simulink model "SIFT-Sysgen"  (R2013a)
settings: Solver=FixedStepDiscrete  SolverMode=SingleTasking  StartTime=0.0  StopTime=10.0  RelTol=1e-3
libraries: xbsIndex_r4 x365, xrbsImage_r4 x64
(part 3 of 10)

== system SIFT-Sysgen/Window Generator ==
  In1 : Inport
  Delay{,1..5} (6 alike) : xbsIndex_r4/Delay  rst=off  infoeditControl=Selection of Reset will increase slice count due to use of real FFs and instead of SRLs  en=off  latency=1  dbl_ovrd=off  reg_retiming=off  block_type=delay
  Virtex Line Buffer : xrbsImage_r4/Virtex Line Buffer  buf_depth=1200  cst=1
  Virtex Line Buffer1 : xrbsImage_r4/Virtex Line Buffer  buf_depth=1200  cst=1
  Out1 : Outport
  Out2 : Outport  Port=2
  Out3 : Outport  Port=3
  Out4 : Outport  Port=4
  Out5 : Outport  Port=5
  Out6 : Outport  Port=6
  Out7 : Outport  Port=7
  Out8 : Outport  Port=8
  Out9 : Outport  Port=9
  wires:
  In1/1 -> Out1/1, Delay/1
  Delay/1 -> Out2/1, Delay1/1
  Delay4/1 -> Out8/1, Delay5/1
  Delay2/1 -> Out5/1, Delay3/1
  Virtex Line Buffer/1 -> Delay4/1, Out7/1
  Virtex Line Buffer1/1 -> Out4/1, Delay2/1
  Delay1/1 -> Virtex Line Buffer1/1, Out3/1
  Delay3/1 -> Virtex Line Buffer/1, Out6/1
  Delay5/1 -> Out9/1

== system SIFT-Sysgen/Window Generator1 ==
  In1 : Inport
  Delay{,1..5} (6 alike) : xbsIndex_r4/Delay  rst=off  infoeditControl=Selection of Reset will increase slice count due to use of real FFs and instead of SRLs  en=off  latency=1  dbl_ovrd=off  reg_retiming=off  block_type=delay
  Virtex Line Buffer : xrbsImage_r4/Virtex Line Buffer  buf_depth=1200  cst=1
  Virtex Line Buffer1 : xrbsImage_r4/Virtex Line Buffer  buf_depth=1200  cst=1
  Out1 : Outport
  Out2 : Outport  Port=2
  Out3 : Outport  Port=3
  Out4 : Outport  Port=4
  Out5 : Outport  Port=5
  Out6 : Outport  Port=6
  Out7 : Outport  Port=7
  Out8 : Outport  Port=8
  Out9 : Outport  Port=9
  wires:
  In1/1 -> Out1/1, Delay/1
  Delay/1 -> Out2/1, Delay1/1
  Delay4/1 -> Out8/1, Delay5/1
  Delay2/1 -> Out5/1, Delay3/1
  Virtex Line Buffer/1 -> Delay4/1, Out7/1
  Virtex Line Buffer1/1 -> Out4/1, Delay2/1
  Delay1/1 -> Virtex Line Buffer1/1, Out3/1
  Delay3/1 -> Virtex Line Buffer/1, Out6/1
  Delay5/1 -> Out9/1

== system SIFT-Sysgen/Window Generator2 ==
  In1 : Inport
  Delay{,1..5} (6 alike) : xbsIndex_r4/Delay  rst=off  infoeditControl=Selection of Reset will increase slice count due to use of real FFs and instead of SRLs  en=off  latency=1  dbl_ovrd=off  reg_retiming=off  block_type=delay
  Virtex Line Buffer : xrbsImage_r4/Virtex Line Buffer  buf_depth=1200  cst=1
  Virtex Line Buffer1 : xrbsImage_r4/Virtex Line Buffer  buf_depth=1200  cst=1
  Out1 : Outport
  Out2 : Outport  Port=2
  Out3 : Outport  Port=3
  Out4 : Outport  Port=4
  Out5 : Outport  Port=5
  Out6 : Outport  Port=6
  Out7 : Outport  Port=7
  Out8 : Outport  Port=8
  Out9 : Outport  Port=9
  wires:
  In1/1 -> Out1/1, Delay/1
  Delay/1 -> Out2/1, Delay1/1
  Delay4/1 -> Out8/1, Delay5/1
  Delay2/1 -> Out5/1, Delay3/1
  Virtex Line Buffer/1 -> Delay4/1, Out7/1
  Virtex Line Buffer1/1 -> Out4/1, Delay2/1
  Delay1/1 -> Virtex Line Buffer1/1, Out3/1
  Delay3/1 -> Virtex Line Buffer/1, Out6/1
  Delay5/1 -> Out9/1

== system SIFT-Sysgen/Window Generator3 ==
  In1 : Inport
  Delay{,1..5} (6 alike) : xbsIndex_r4/Delay  rst=off  infoeditControl=Selection of Reset will increase slice count due to use of real FFs and instead of SRLs  en=off  latency=1  dbl_ovrd=off  reg_retiming=off  block_type=delay
  Virtex Line Buffer : xrbsImage_r4/Virtex Line Buffer  buf_depth=1200  cst=1
  Virtex Line Buffer1 : xrbsImage_r4/Virtex Line Buffer  buf_depth=1200  cst=1
  Out1 : Outport
  Out2 : Outport  Port=2
  Out3 : Outport  Port=3
  Out4 : Outport  Port=4
  Out5 : Outport  Port=5
  Out6 : Outport  Port=6
  Out7 : Outport  Port=7
  Out8 : Outport  Port=8
  Out9 : Outport  Port=9
  wires:
  In1/1 -> Out1/1, Delay/1
  Delay/1 -> Out2/1, Delay1/1
  Delay4/1 -> Out8/1, Delay5/1
  Delay2/1 -> Out5/1, Delay3/1
  Virtex Line Buffer/1 -> Delay4/1, Out7/1
  Virtex Line Buffer1/1 -> Out4/1, Delay2/1
  Delay1/1 -> Virtex Line Buffer1/1, Out3/1
  Delay3/1 -> Virtex Line Buffer/1, Out6/1
  Delay5/1 -> Out9/1

== system SIFT-Sysgen/Window Generator4 ==
  In1 : Inport
  Delay{,1..5} (6 alike) : xbsIndex_r4/Delay  rst=off  infoeditControl=Selection of Reset will increase slice count due to use of real FFs and instead of SRLs  en=off  latency=1  dbl_ovrd=off  reg_retiming=off  block_type=delay
  Virtex Line Buffer : xrbsImage_r4/Virtex Line Buffer  buf_depth=1200  cst=1
  Virtex Line Buffer1 : xrbsImage_r4/Virtex Line Buffer  buf_depth=1200  cst=1
  Out1 : Outport
  Out2 : Outport  Port=2
  Out3 : Outport  Port=3
  Out4 : Outport  Port=4
  Out5 : Outport  Port=5
  Out6 : Outport  Port=6
  Out7 : Outport  Port=7
  Out8 : Outport  Port=8
  Out9 : Outport  Port=9
  wires:
  In1/1 -> Out1/1, Delay/1
  Delay/1 -> Out2/1, Delay1/1
  Delay4/1 -> Out8/1, Delay5/1
  Delay2/1 -> Out5/1, Delay3/1
  Virtex Line Buffer/1 -> Delay4/1, Out7/1
  Virtex Line Buffer1/1 -> Out4/1, Delay2/1
  Delay1/1 -> Virtex Line Buffer1/1, Out3/1
  Delay3/1 -> Virtex Line Buffer/1, Out6/1
  Delay5/1 -> Out9/1
